simulink model "BreakerFeederFault"  (R2019a)
settings: Solver=ode1  StartTime=0.0  StopTime=2.5  FixedStep=Ts_Power  RelTol=1e-3
PostLoadFcn:
  | %% Init for wind PnO models - global system parameters
  | OVERRIDE_SSN_MEMORY_LIMIT=1;
  | Ts=50e-6;
  | % Ts=50e-10;
  | Ts_Power=Ts;
  | Ts_Control=2*Ts;
  | freq = 50;
  | Fnom=freq;
  | Vac=400e3;
InitFcn:
  | %% Init for wind PnO models - global system parameters
  | OVERRIDE_SSN_MEMORY_LIMIT=1;
  | Ts=50e-6;
  | % Ts=50e-10;
  | Ts_Power=Ts;
  | Ts_Control=2*Ts;
  | freq = 50;
  | Fnom=freq;
  | Vac=225e3;
values from neighbouring files (symbols this model uses):
  ohl_posCap = (0.01e-006)*12    (= 1.2e-07)    [variable.m]
  ohl_posInd = (1.15e-3)/12    (= 9.58333333333e-05)    [variable.m]
  ohl_posR = 0.069/12    (= 0.00575)    [variable.m]
  ohl_zeroCap = (0.004e-006)*12    (= 4.8e-08)    [variable.m]
  ohl_zeroInd = (2.86e-3)/12    (= 0.000238333333333)    [variable.m]
  ohl_zeroR = 0.1725/12    (= 0.014375)    [variable.m]
  sub_Ind = compensate_power    (= 870283996.897)    [variable.m]
  sub_posCap = sub_posCap*6    (= 9.6e-07)    [variable.m]
  sub_posInd = sub_posInd/6    (= 0.000233333333333)    [variable.m]
  sub_posR = sub_posR/6    (= 0.006)    [variable.m]
  sub_zeroCap = sub_zeroCap*6    (= 3.84e-07)    [variable.m]
  sub_zeroInd = sub_zeroInd/6    (= 0.000583333333333)    [variable.m]
  sub_zeroR = sub_zeroR/6    (= 0.015)    [variable.m]
  transfo_L1 = 0.05999374    [variable.m]
  transfo_L2 = 0.05999374    [variable.m]
  transfo_R1 = 0.000866667    [variable.m]
  transfo_R2 = 0.00086667    [variable.m]
undefined symbols (not defined in the file or in its folder): D1, D11, Delta, den, DiscIntNeverNeededParam, dx, find_system, gcbh, num, out_Buses, out_WindFarms, sps_rtmsupport
libraries: powerlib x209, simulink x96, powerlib_meascontrol x96, elements x52, eeSinusoidalMeasurement x51, simulink_extras x42, spsVIMeasurementModel x36, eePowerMeasurement x16
(part 8 of 24)

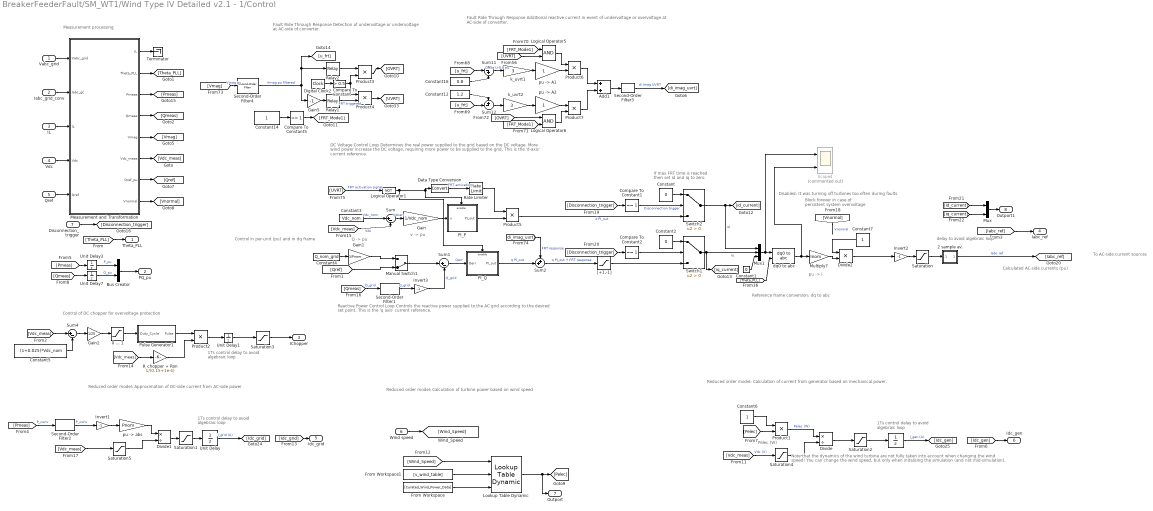
== system BreakerFeederFault/SM_WT1/Wind Type IV Detailed v2.1 - 1/Control ==
  note: Pelec (W)
  note: Note that the dynamics of the wind turbine are not fully taken into account when changing the wind speed! You can change the wind speed, but only when initalising the simulation (and not mid-simulation).
  note: 1Ts control delay to
      | avoid algebraic loop
  note: Reduced order model: Calculation of turbine power based on wind speed
  note: Block forever in case of
      | persistent system overvoltage
  note: 1Ts control delay to
      | avoid algebraic loop
  note: delay to avoid
      |  algebraic loop
  note: Reduced order model: Calculation of current from generator based on mechanical power.
  note: Reduced order model: Approximation of DC-side current from AC-side power
  note: 1Ts control delay to
      | avoid algebraic loop
  note: Reference frame conversion: dq to abc
  note: Control in per-unit (pu) and in dq frame
  note: v -> pu
  note: Reactive Power Control Loop
      | Controls the reactive power supplied to the AC grid according to the desired set point. This is the 'q axis' current reference.
  note: DC Voltage Control Loop
      | Determines the real power supplied to the grid based on the DC voltage. More wind power increase the DC voltage, requiring more power to be supplied to the grid. This is the 'd-axis' current reference.
  note: To AC-side current sources
  note: Q -> pu
  note: pu -> i
  note: Calculated AC-side currents (pu)
  note: Fault Ride Through Response
      | Detection of undervoltage or undervoltage at AC-side of converter.
  note: Fault Ride Through Response
      | Additional reactive current in event of undervoltage or overvoltage at AC-side of converter.
  note: Control of DC chopper for overvoltage protection
  note: Measurement processing
  note: If max FRT time is reached
      | then set id and iq to zero
  note: Disabled: It was turning off turbines too often during faults
  Vabc_grid : Inport
  Iabc_grid_conv : Inport  Port=2
  IL : Inport  Port=3
  Vdc : Inport  Port=4
  Qref : Inport  Port=5
  Wind speed : Inport  Port=6
  Disconnection_trigger : Inport  Port=7
  " " : UnitDelay  SampleTime=-1  HasFrameUpgradeWarning=on
  0 ... 1 : Saturate  UpperLimit=1  LowerLimit=0
  2 sample av. : Subsystem  mask{Init_value=0, Ts=Ts}
      mask prompts: Init_value "Initial value:"; Ts "Sample time (Ts):"
  Add1 : Sum
  Bus Creator : BusCreator  Inputs=2
  Compare To Constant : simulink/Logic and Bit Operations/Compare To Constant  relop=>  const=0.5  OutDataTypeStr=boolean
  Compare To Constant1 : simulink/Logic and Bit Operations/Compare To Constant  relop===  const=1  OutDataTypeStr=boolean
  Compare To Constant2 : simulink/Logic and Bit Operations/Compare To Constant  relop===  const=1  OutDataTypeStr=boolean
  Compare To Constant5 : simulink/Logic and Bit Operations/Compare To Constant  relop===  const=1  OutDataTypeStr=boolean
  Constant : Constant  Value=0
  Constant1 : Constant  Value=0  OutDataTypeStr=Inherit: Inherit via back propagation
  Constant12 : Constant  Value=1.2  SampleTime=Ts
  Constant14 : Constant  SampleTime=Ts
  Constant16 : Constant  Value=0.8  SampleTime=Ts
  Constant2 : Constant  Value=0
  Constant3 : Constant  Value=Vdc_nom
  Constant4 : Constant  Value=Q_nom_grid
  Constant5 : Constant  Value=(1+0.025)*Vdc_nom  SampleTime=Ts
  Constant6 : Constant
  Constant7 : Constant
  Data Type Conversion : DataTypeConversion
  Digital Clock2 : DigitalClock  SampleTime=Ts
  Divide : Product  Inputs=*/
  Divide1 : Product  Inputs=*/
  Divide2 : Product  Inputs=**
  From Workspace : FromWorkspace  VariableName=[Curated_Wind_Power_Data]  SampleTime=0
  From Workspace1 : FromWorkspace  VariableName=[v_wind_table]  SampleTime=0
  Gain : Gain  Gain=1/Vdc_nom
  Gain1 : Gain  Gain=1/Pnom
  Gain2 : Gain  Gain=1/20
  Gain5 : Gain  Gain=-1
  Invert1 : Gain  Gain=-1
  Invert2 : Gain  Gain=-1
  Invert3 : Gain  Gain=-1
  Logical Operator1 : Logic  Operator=NOT  AllPortsSameDT=off  OutDataTypeStr=boolean
  Logical Operator5 : Logic  AllPortsSameDT=off  OutDataTypeStr=boolean
  Logical Operator6 : Logic  AllPortsSameDT=off  OutDataTypeStr=boolean
  Lookup Table Dynamic : simulink/Lookup Tables/Lookup Table Dynamic  LookUpMeth=Interpolation-Use End Values  OutDataType=fixdt('double')  OutScaling=[]  OutputDataTypeScalingMode=Specify via dialog  OutDataTypeStr=double  DoSatur=off
  Manual Switch1 : ManualSwitch  CurrentSetting=0
  Measurement and Transformation : Subsystem
  Multiply7 : Gain  Gain=Inom
  Mux : Mux  Inputs=2
  Mux1 : Mux  Inputs=3
  PI_P : Subsystem
  PI_Q : Subsystem
  Product{1..7} (7 alike) : Product
  Pulse Generator1 : Subsystem  mask{Freq_sawtooth=Freq_sawtooth, Ts=Ts}
      mask prompts: Freq_sawtooth "Frequency of the carrier (sawtooth signal) (Hz):"; Ts "Sample time (Ts) (s):"
  R_chopper + Ron : Gain  Gain=1/(0.15+1e-4)
  Rate Limiter : RateLimiter  RisingSlewLimit=200  FallingSlewLimit=-100  SampleTimeMode=inherited
  Relay1 : Relay  OnSwitchValue=-(0.7)  OffSwitchValue=-(0.8 + 0.05)  OutDataTypeStr=Inherit: Inherit via back propagation
  Relay2 : Relay  OnSwitchValue=1.2 + 0.05  OffSwitchValue=1.2 - 0.05  OutDataTypeStr=Inherit: Inherit via back propagation
  Saturation : Saturate  UpperLimit=1e6  LowerLimit=-1e6
  Saturation1 : Saturate  UpperLimit=1e6  LowerLimit=-1e6
  Saturation2 : Saturate  UpperLimit=1e6  LowerLimit=-1e6
  Saturation3 : Saturate  UpperLimit=10e3  LowerLimit=-10e3
  Saturation4 : Saturate  UpperLimit=1e6  LowerLimit=10
  Saturation5 : Saturate  UpperLimit=1e6  LowerLimit=10
  Scope4 : Scope  Commented=on  NumInputPorts=2
  Second-Order Filter1 : powerlib_meascontrol/Filters/Second-Order Filter  FilterType=Lowpass  Fo=50  Zeta=0.707  Ts=Ts  Initialize=off  Vac_Init="[0,  0,  60]"  Vdc_Init=0  PlotResponse=off  FreqRange=[0, 500, 1]
      settings: SourceProductBaseCode=PS
  Second-Order Filter2 : powerlib_meascontrol/Filters/Second-Order Filter  FilterType=Lowpass  Fo=50  Zeta=0.707  Ts=Ts  Initialize=off  Vac_Init="[0,  0,  60]"  Vdc_Init=0  PlotResponse=off  FreqRange=[0, 500, 1]
      settings: SourceProductBaseCode=PS
  Second-Order Filter3 : powerlib_meascontrol/Filters/Second-Order Filter  FilterType=Lowpass  Fo=1e3  Zeta=0.707  Ts=Ts  Initialize=off  Vac_Init="[0,  0,  60]"  Vdc_Init=0  PlotResponse=off  FreqRange=[0, 500, 1]
      settings: SourceProductBaseCode=PS
  Second-Order Filter4 : powerlib_meascontrol/Filters/Second-Order Filter  FilterType=Lowpass  Fo=100  Zeta=0.707  Ts=Ts  Initialize=off  Vac_Init="[0,  0,  60]"  Vdc_Init=0  PlotResponse=off  FreqRange=[0, 500, 1]
      settings: SourceProductBaseCode=PS
  Sum : Sum  Inputs=|+-
  Sum1 : Sum  Inputs=|+-
  Sum11 : Sum  Inputs=|-+
  Sum12 : Sum  Inputs=+-|
  Sum2 : Sum  Inputs=++|
  Sum4 : Sum  Inputs=|+-
  Switch1 : Switch  Criteria=u2 > Threshold
  Switch2 : Switch  Criteria=u2 > Threshold
  Terminator : Terminator
  Unit Delay : UnitDelay  SampleTime=-1  HasFrameUpgradeWarning=on
  Unit Delay1 : UnitDelay  SampleTime=Ts  HasFrameUpgradeWarning=on
  Unit Delay3 : UnitDelay  SampleTime=Ts  HasFrameUpgradeWarning=on
  Unit Delay7 : UnitDelay  SampleTime=Ts  HasFrameUpgradeWarning=on
  "[+1,-1]" : Saturate  UpperLimit=1  LowerLimit=-1
  dq0 to abc : powerlib_meascontrol/Transformations/dq0 to abc  Alignment=90 degrees behind phase A axis
  k_uvrt1 : Gain  Gain=3
  k_uvrt2 : Gain  Gain=3
  "pu -> A1" : Gain
  "pu -> A2" : Gain
  "pu -> abs" : Gain  Gain=Pnom
  Theta_PLL : Outport  VectorParamsAs1DForOutWhenUnconnected=on
  PQ_pu : Outport  Port=2  VectorParamsAs1DForOutWhenUnconnected=on
  IChopper : Outport  Port=3  VectorParamsAs1DForOutWhenUnconnected=on
  Iabc_ref : Outport  Port=4  VectorParamsAs1DForOutWhenUnconnected=on
  Idc_grid : Outport  Port=5  VectorParamsAs1DForOutWhenUnconnected=on
  Idc_gen : Outport  Port=6  VectorParamsAs1DForOutWhenUnconnected=on
  Outport : Outport  Port=7  VectorParamsAs1DForOutWhenUnconnected=on
  Outport1 : Outport  Port=8  VectorParamsAs1DForOutWhenUnconnected=on
  wires:
  Constant7/1 -> Divide2/1
  Disconnection_trigger/1 -> [Disconnection_trigger]
  Mux/1 -> Outport1/1
  [iq_current] -> Mux/2
  [id_current] -> Mux/1
  Compare To Constant2/1 -> Switch1/2
  [Disconnection_trigger] -> Compare To Constant2/1
  Compare To Constant1/1 -> Switch2/2  "Disconnection trigger"
  [Disconnection_trigger] -> Compare To Constant1/1
  "[+1,-1]"/1 -> Switch1/3
  Constant2/1 -> Switch1/1
  Product5/1 -> Switch2/3  "d PI_out"
  Constant/1 -> Switch2/1
  Switch1/1 -> Mux1/2, [iq_current]  "iq"
  Switch2/1 -> [id_current], Mux1/1  "id"
  From Workspace/1 -> Lookup Table Dynamic/3
  From Workspace1/1 -> Lookup Table Dynamic/2
  [Wind_Speed] -> Lookup Table Dynamic/1
  Lookup Table Dynamic/1 -> [Pelec], Outport/1
  Logical Operator1/1 -> PI_Q/Enable, PI_P/Enable, Data Type Conversion/1
  [UVRT] -> Logical Operator1/1  "FRT activation signal"
  [di_imag_uvrt] -> Sum2/1  "FRT response"
  Sum2/1 -> "[+1,-1]"/1  "q PI_out + FRT response"
  Second-Order Filter3/1 -> [di_imag_uvrt]  "di Imag UVRT"
  2 sample av./1(out) -> [Iabc_ref]  "Iabc ref"
  [Iabc_ref] -> Iabc_ref/1
  Product6/1 -> Add1/1
  " "/1 -> [Idc_gen]  "I_gen (A)"
  Product1/1 -> Divide/1  "Pelec (W)"
  [Pelec] -> Product1/2
  [Idc_gen] -> Idc_gen/1
  Constant6/1 -> Product1/1
  [Vdc_meas] -> Saturation4/1  "Vdc (V)"
  Saturation2/1 -> " "/1
  Divide/1 -> Saturation2/1
  Saturation4/1 -> Divide/2
  Wind speed/1 -> [Wind_Speed]
  [Vnormal] -> ?  "Vnormal"
  Divide2/1 -> Invert2/1
  Measurement and Transformation/8(Vnormal) -> [Vnormal]
  PI_Q/1(PI_out) -> Sum2/2  "q PI_out"
  Saturation5/1 -> Divide1/2
  Saturation1/1 -> Unit Delay/1
  Saturation/1 -> 2 sample av./1(in)
  PI_P/1(PI_out) -> Product5/2
  Gain/1 -> PI_P/1(u)
  Rate Limiter/1 -> Product5/1
  Constant4/1 -> Gain1/1
  [Pmeas] -> Second-Order Filter2/1  "P_conv"
  [Qmeas] -> Second-Order Filter1/1  "Q_grid"
  Second-Order Filter1/1 -> Invert3/1  "Q_grid"
  Saturation3/1 -> IChopper/1
  Invert2/1 -> Saturation/1
  [Idc_grid] -> Idc_grid/1
  [Vdc_meas] -> Saturation5/1
  Second-Order Filter2/1 -> Invert1/1  "P_conv"
  Unit Delay/1 -> [Idc_grid]  "I_grid (A)"
  Divide1/1 -> Saturation1/1
  Invert1/1 -> "pu -> abs"/1
  "pu -> abs"/1 -> Divide1/1
  Measurement and Transformation/7(Qref_pu) -> [Qref]
  Sum/1 -> Gain/1  "Vdcerr"
  [Theta_PLL] -> dq0 to abc/2
  Sum1/1 -> PI_Q/1(Qerr)  "Qerr"
  Constant3/1 -> Sum/1  "Vdc_nom"
  Invert3/1 -> Sum1/2  "Q_grid"
  [Vdc_meas] -> Sum/2  "Vdc"
  Mux1/1 -> dq0 to abc/1, Scope4/1
  Manual Switch1/1 -> Sum1/1
  dq0 to abc/1 -> Multiply7/1, Scope4/2
  Constant1/1 -> Mux1/3
  Data Type Conversion/1 -> Rate Limiter/1  "FRT activation"
  Gain1/1 -> Manual Switch1/1
  Multiply7/1 -> Divide2/2
  [Qref] -> Manual Switch1/2
  Relay1/1 -> Product4/2  "FRT triggered"
  "pu -> A2"/1 -> Product7/1
  [FRT_Mode1] -> Logical Operator5/1
  k_uvrt1/1 -> "pu -> A1"/1
  [FRT_Mode1] -> Logical Operator6/2
  Sum12/1 -> k_uvrt2/1
  [Vmag] -> Second-Order Filter4/1  "Vmag pu"
  k_uvrt2/1 -> "pu -> A2"/1
  Gain5/1 -> Relay1/1
  [OVRT] -> Logical Operator6/1
  Logical Operator5/1 -> Product6/1
  Sum11/1 -> k_uvrt1/1  "Delta U-0.8 pu"
  Logical Operator6/1 -> Product7/2
  Second-Order Filter4/1 -> Gain5/1, Relay2/1, [u_frt]  "Vmag pu filtered"
  Constant16/1 -> Sum11/2
  Product3/1 -> [OVRT]
  Digital Clock2/1 -> Compare To Constant/1
  Add1/1 -> Second-Order Filter3/1
  Product4/1 -> [UVRT]
  Relay2/1 -> Product3/1
  Product7/1 -> Add1/2
  "pu -> A1"/1 -> Product6/2
  Compare To Constant/1 -> Product3/2, Product4/1
  [UVRT] -> Logical Operator5/2
  [u_frt] -> Sum12/2
  Constant12/1 -> Sum12/1
  Compare To Constant5/1 -> [FRT_Mode1]
  [u_frt] -> Sum11/1
  Constant14/1 -> Compare To Constant5/1
  Unit Delay1/1 -> Saturation3/1
  Pulse Generator1/1(Pulse) -> Product2/1
  [Vdc_meas] -> R_chopper + Ron/1
  Product2/1 -> Unit Delay1/1
  R_chopper + Ron/1 -> Product2/2
  Measurement and Transformation/6(Vdc_meas) -> [Vdc_meas]
  0 ... 1/1 -> Pulse Generator1/1(Duty_Cycle)
  Gain2/1 -> 0 ... 1/1
  Sum4/1 -> Gain2/1
  [Vdc_meas] -> Sum4/1
  Constant5/1 -> Sum4/2
  Measurement and Transformation/5(Vmag) -> [Vmag]
  Measurement and Transformation/4(Qmeas) -> [Qmeas]
  Measurement and Transformation/3(Pmeas) -> [Pmeas]
  [Theta_PLL] -> Theta_PLL/1
  Vabc_grid/1 -> Measurement and Transformation/1(Vabc_grid)
  Iabc_grid_conv/1 -> Measurement and Transformation/2(Iabc_gc)
  IL/1 -> Measurement and Transformation/3(IL)
  Qref/1 -> Measurement and Transformation/5(Qref)
  Measurement and Transformation/2(Theta_PLL) -> [Theta_PLL]
  Measurement and Transformation/1("IL ") -> Terminator/1
  Vdc/1 -> Measurement and Transformation/4(Vdc)
  [Pmeas] -> Unit Delay3/1
  [Qmeas] -> Unit Delay7/1
  Unit Delay7/1 -> Bus Creator/2  "Q_pu"
  Unit Delay3/1 -> Bus Creator/1  "P_pu"
  Bus Creator/1 -> PQ_pu/1

== system BreakerFeederFault/SM_WT1/Wind Type IV Detailed v2.1 - 2/AC fault ride though characteristic ==
  note: If more than X seconds under
      | FRT then disconnection message
  Va pu mag : Inport
  I 3ph pu : Inport  Port=2
  Compare To Constant : simulink/Logic and Bit Operations/Compare To Constant  relop=>=  const=Fault_Base_Duration_time_FRT  OutDataTypeStr=boolean
  Compare To Constant1 : simulink/Logic and Bit Operations/Compare To Constant  relop=<  const=0.2  OutDataTypeStr=boolean
  Compare To Constant2 : simulink/Logic and Bit Operations/Compare To Constant  relop=<  const=0.2  OutDataTypeStr=boolean
  Compare To Constant3 : simulink/Logic and Bit Operations/Compare To Constant  relop=<  const=0.5  OutDataTypeStr=boolean
  Constant : Constant  Value=0  SampleTime=Ts
  Constant1 : Constant  SampleTime=Ts
  Constant2 : Constant  Value=0  SampleTime=Ts
  Constant3 : Constant  Value=0
  Constant4 : Constant  Value=0
  Constant5 : Constant  Value=0
  Constant6 : Constant  Value=0.9  SampleTime=Ts
  Data Type Conversion : DataTypeConversion  OutDataTypeStr=double
  Digital Clock{1..4} (4 alike) : DigitalClock  SampleTime=Ts
  Discrete-Time Integrator : DiscreteIntegrator  ExternalReset=rising  SampleTime=Ts  ICPrevOutput=DiscIntNeverNeededParam  ICPrevScaledInput=DiscIntNeverNeededParam
  Memory : Memory
  MinMax : MinMax  Function=max
  MinMax Running Resettable : simulink/Math Operations/MinMax Running Resettable  Function=max  vinit=0.0
  MinMax Running Resettable1 : simulink/Math Operations/MinMax Running Resettable  Function=min  vinit=1
  MinMax Running Resettable2 : simulink/Math Operations/MinMax Running Resettable  Function=max  vinit=0.0
  MinMax1 : MinMax  Function=max
  MinMax2 : MinMax
  NOT : Logic  Operator=NOT  AllPortsSameDT=off  OutDataTypeStr=boolean
  OR : Logic  Operator=OR  AllPortsSameDT=off  OutDataTypeStr=boolean
  Relational Operator : RelationalOperator  Operator=<  OutDataTypeStr=boolean  RndMeth=Simplest
  "Sinusoidal Measurement (PLL, Three-Phase)1" : eeSinusoidalMeasurement/Sinusoidal Measurement (PLL, Three-Phase)  Kp_LF=200  Ki_LF=2000  F0=freq  Theta0=0  Ts=Ts
      settings: SourceProductBaseCode=PS
  Switch1 : Switch  Criteria=u2 > Threshold
  Switch2 : Switch  Criteria=u2 > Threshold
  Switch3 : Switch  Criteria=u2 > Threshold
  Terminator : Terminator
  Terminator1 : Terminator
  Triggered Subsystem : Subsystem  TreatAsAtomicUnit=on
  Disconnection_trigger : Outport  VectorParamsAs1DForOutWhenUnconnected=on
  Time_under_FRT : Outport  Port=2  VectorParamsAs1DForOutWhenUnconnected=on
  Min_voltage : Outport  Port=3  VectorParamsAs1DForOutWhenUnconnected=on
  Max_current : Outport  Port=4  VectorParamsAs1DForOutWhenUnconnected=on
  Time_trigger_FRT : Outport  Port=5  VectorParamsAs1DForOutWhenUnconnected=on
  wires:
  Constant6/1 -> Relational Operator/2
  Discrete-Time Integrator/1 -> Compare To Constant/1, MinMax/1  "Integrator output"
  Digital Clock1/1 -> Compare To Constant3/1
  Relational Operator/1 -> Switch2/3
  Compare To Constant3/1 -> Switch2/2
  Constant/1 -> Switch2/1
  Switch2/1 -> NOT/1, Discrete-Time Integrator/1  "Va comparison to Vgrid"
  NOT/1 -> Discrete-Time Integrator/2
  OR/1 -> Triggered Subsystem/Trigger, Data Type Conversion/1, Memory/1  "Disconnection_Trigger"
  Compare To Constant/1 -> OR/2
  Memory/1 -> OR/1
  MinMax/1 -> MinMax Running Resettable/1
  MinMax Running Resettable/1 -> Time_under_FRT/1
  Va pu mag/1 -> Relational Operator/1, Switch3/3
  MinMax1/1 -> MinMax Running Resettable2/1
  MinMax Running Resettable2/1 -> Max_current/1
  I 3ph pu/1 -> "Sinusoidal Measurement (PLL, Three-Phase)1"/1
  "Sinusoidal Measurement (PLL, Three-Phase)1"/3 -> Switch1/3  "Vabc_pu_mag"
  "Sinusoidal Measurement (PLL, Three-Phase)1"/2 -> Terminator/1
  "Sinusoidal Measurement (PLL, Three-Phase)1"/1 -> Terminator1/1
  MinMax Running Resettable1/1 -> Min_voltage/1
  Compare To Constant1/1 -> Switch3/2
  Constant1/1 -> Switch3/1
  Digital Clock2/1 -> Compare To Constant1/1
  Digital Clock3/1 -> Triggered Subsystem/1(In1)
  Triggered Subsystem/1(Time_trigger_FRT) -> Time_trigger_FRT/1
  Digital Clock4/1 -> Compare To Constant2/1
  Constant2/1 -> Switch1/1
  Compare To Constant2/1 -> Switch1/2
  Switch1/1 -> MinMax1/1
  Switch3/1 -> MinMax2/1
  MinMax2/1 -> MinMax Running Resettable1/1
  Constant3/1 -> MinMax Running Resettable/2
  Constant4/1 -> MinMax Running Resettable1/2
  Constant5/1 -> MinMax Running Resettable2/2
  Data Type Conversion/1 -> Disconnection_trigger/1

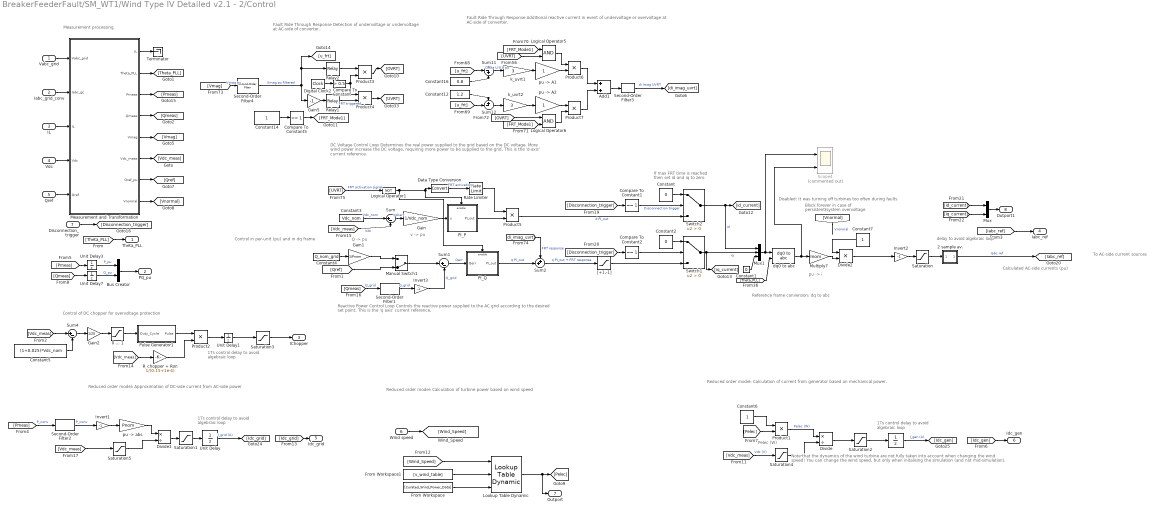
== system BreakerFeederFault/SM_WT1/Wind Type IV Detailed v2.1 - 2/Control ==
  note: Disabled: It was turning off turbines too often during faults
  note: If max FRT time is reached
      | then set id and iq to zero
  note: Measurement processing
  note: Control of DC chopper for overvoltage protection
  note: Fault Ride Through Response
      | Additional reactive current in event of undervoltage or overvoltage at AC-side of converter.
  note: Fault Ride Through Response
      | Detection of undervoltage or undervoltage at AC-side of converter.
  note: Calculated AC-side currents (pu)
  note: pu -> i
  note: Q -> pu
  note: To AC-side current sources
  note: DC Voltage Control Loop
      | Determines the real power supplied to the grid based on the DC voltage. More wind power increase the DC voltage, requiring more power to be supplied to the grid. This is the 'd-axis' current reference.
  note: Reactive Power Control Loop
      | Controls the reactive power supplied to the AC grid according to the desired set point. This is the 'q axis' current reference.
  note: v -> pu
  note: Control in per-unit (pu) and in dq frame
  note: Reference frame conversion: dq to abc
  note: 1Ts control delay to
      | avoid algebraic loop
  note: Reduced order model: Approximation of DC-side current from AC-side power
  note: Reduced order model: Calculation of current from generator based on mechanical power.
  note: delay to avoid
      |  algebraic loop
  note: 1Ts control delay to
      | avoid algebraic loop
  note: Block forever in case of
      | persistent system overvoltage
  note: Reduced order model: Calculation of turbine power based on wind speed
  note: 1Ts control delay to
      | avoid algebraic loop
  note: Note that the dynamics of the wind turbine are not fully taken into account when changing the wind speed! You can change the wind speed, but only when initalising the simulation (and not mid-simulation).
  note: Pelec (W)
  Vabc_grid : Inport
  Iabc_grid_conv : Inport  Port=2
  IL : Inport  Port=3
  Vdc : Inport  Port=4
  Qref : Inport  Port=5
  Wind speed : Inport  Port=6
  Disconnection_trigger : Inport  Port=7
  " " : UnitDelay  SampleTime=-1  HasFrameUpgradeWarning=on
  0 ... 1 : Saturate  UpperLimit=1  LowerLimit=0
  2 sample av. : Subsystem  mask{Init_value=0, Ts=Ts}
      mask prompts: Init_value "Initial value:"; Ts "Sample time (Ts):"
  Add1 : Sum
  Bus Creator : BusCreator  Inputs=2
  Compare To Constant : simulink/Logic and Bit Operations/Compare To Constant  relop=>  const=0.5  OutDataTypeStr=boolean
  Compare To Constant1 : simulink/Logic and Bit Operations/Compare To Constant  relop===  const=1  OutDataTypeStr=boolean
  Compare To Constant2 : simulink/Logic and Bit Operations/Compare To Constant  relop===  const=1  OutDataTypeStr=boolean
  Compare To Constant5 : simulink/Logic and Bit Operations/Compare To Constant  relop===  const=1  OutDataTypeStr=boolean
  Constant : Constant  Value=0
  Constant1 : Constant  Value=0  OutDataTypeStr=Inherit: Inherit via back propagation
  Constant12 : Constant  Value=1.2  SampleTime=Ts
  Constant14 : Constant  SampleTime=Ts
  Constant16 : Constant  Value=0.8  SampleTime=Ts
  Constant2 : Constant  Value=0
  Constant3 : Constant  Value=Vdc_nom
  Constant4 : Constant  Value=Q_nom_grid
  Constant5 : Constant  Value=(1+0.025)*Vdc_nom  SampleTime=Ts
  Constant6 : Constant
  Constant7 : Constant
  Data Type Conversion : DataTypeConversion
  Digital Clock2 : DigitalClock  SampleTime=Ts
  Divide : Product  Inputs=*/
  Divide1 : Product  Inputs=*/
  Divide2 : Product  Inputs=**
  From Workspace : FromWorkspace  VariableName=[Curated_Wind_Power_Data]  SampleTime=0
  From Workspace1 : FromWorkspace  VariableName=[v_wind_table]  SampleTime=0
  Gain : Gain  Gain=1/Vdc_nom
  Gain1 : Gain  Gain=1/Pnom
  Gain2 : Gain  Gain=1/20
  Gain5 : Gain  Gain=-1
  Invert1 : Gain  Gain=-1
  Invert2 : Gain  Gain=-1
  Invert3 : Gain  Gain=-1
  Logical Operator1 : Logic  Operator=NOT  AllPortsSameDT=off  OutDataTypeStr=boolean
  Logical Operator5 : Logic  AllPortsSameDT=off  OutDataTypeStr=boolean
  Logical Operator6 : Logic  AllPortsSameDT=off  OutDataTypeStr=boolean
  Lookup Table Dynamic : simulink/Lookup Tables/Lookup Table Dynamic  LookUpMeth=Interpolation-Use End Values  OutDataType=fixdt('double')  OutScaling=[]  OutputDataTypeScalingMode=Specify via dialog  OutDataTypeStr=double  DoSatur=off
  Manual Switch1 : ManualSwitch  CurrentSetting=0
  Measurement and Transformation : Subsystem
  Multiply7 : Gain  Gain=Inom
  Mux : Mux  Inputs=2
  Mux1 : Mux  Inputs=3
  PI_P : Subsystem
  PI_Q : Subsystem
  Product{1..7} (7 alike) : Product
  Pulse Generator1 : Subsystem  mask{Freq_sawtooth=Freq_sawtooth, Ts=Ts}
      mask prompts: Freq_sawtooth "Frequency of the carrier (sawtooth signal) (Hz):"; Ts "Sample time (Ts) (s):"
  R_chopper + Ron : Gain  Gain=1/(0.15+1e-4)
  Rate Limiter : RateLimiter  RisingSlewLimit=200  FallingSlewLimit=-100  SampleTimeMode=inherited
  Relay1 : Relay  OnSwitchValue=-(0.7)  OffSwitchValue=-(0.8 + 0.05)  OutDataTypeStr=Inherit: Inherit via back propagation
  Relay2 : Relay  OnSwitchValue=1.2 + 0.05  OffSwitchValue=1.2 - 0.05  OutDataTypeStr=Inherit: Inherit via back propagation
  Saturation : Saturate  UpperLimit=1e6  LowerLimit=-1e6
  Saturation1 : Saturate  UpperLimit=1e6  LowerLimit=-1e6
  Saturation2 : Saturate  UpperLimit=1e6  LowerLimit=-1e6
  Saturation3 : Saturate  UpperLimit=10e3  LowerLimit=-10e3
  Saturation4 : Saturate  UpperLimit=1e6  LowerLimit=10
  Saturation5 : Saturate  UpperLimit=1e6  LowerLimit=10
  Scope4 : Scope  Commented=on  NumInputPorts=2
  Second-Order Filter1 : powerlib_meascontrol/Filters/Second-Order Filter  FilterType=Lowpass  Fo=50  Zeta=0.707  Ts=Ts  Initialize=off  Vac_Init="[0,  0,  60]"  Vdc_Init=0  PlotResponse=off  FreqRange=[0, 500, 1]
      settings: SourceProductBaseCode=PS
  Second-Order Filter2 : powerlib_meascontrol/Filters/Second-Order Filter  FilterType=Lowpass  Fo=50  Zeta=0.707  Ts=Ts  Initialize=off  Vac_Init="[0,  0,  60]"  Vdc_Init=0  PlotResponse=off  FreqRange=[0, 500, 1]
      settings: SourceProductBaseCode=PS
  Second-Order Filter3 : powerlib_meascontrol/Filters/Second-Order Filter  FilterType=Lowpass  Fo=1e3  Zeta=0.707  Ts=Ts  Initialize=off  Vac_Init="[0,  0,  60]"  Vdc_Init=0  PlotResponse=off  FreqRange=[0, 500, 1]
      settings: SourceProductBaseCode=PS
  Second-Order Filter4 : powerlib_meascontrol/Filters/Second-Order Filter  FilterType=Lowpass  Fo=100  Zeta=0.707  Ts=Ts  Initialize=off  Vac_Init="[0,  0,  60]"  Vdc_Init=0  PlotResponse=off  FreqRange=[0, 500, 1]
      settings: SourceProductBaseCode=PS
  Sum : Sum  Inputs=|+-
  Sum1 : Sum  Inputs=|+-
  Sum11 : Sum  Inputs=|-+
  Sum12 : Sum  Inputs=+-|
  Sum2 : Sum  Inputs=++|
  Sum4 : Sum  Inputs=|+-
  Switch1 : Switch  Criteria=u2 > Threshold
  Switch2 : Switch  Criteria=u2 > Threshold
  Terminator : Terminator
  Unit Delay : UnitDelay  SampleTime=-1  HasFrameUpgradeWarning=on
  Unit Delay1 : UnitDelay  SampleTime=Ts  HasFrameUpgradeWarning=on
  Unit Delay3 : UnitDelay  SampleTime=Ts  HasFrameUpgradeWarning=on
  Unit Delay7 : UnitDelay  SampleTime=Ts  HasFrameUpgradeWarning=on
  "[+1,-1]" : Saturate  UpperLimit=1  LowerLimit=-1
  dq0 to abc : powerlib_meascontrol/Transformations/dq0 to abc  Alignment=90 degrees behind phase A axis
  k_uvrt1 : Gain  Gain=3
  k_uvrt2 : Gain  Gain=3
  "pu -> A1" : Gain
  "pu -> A2" : Gain
  "pu -> abs" : Gain  Gain=Pnom
  Theta_PLL : Outport  VectorParamsAs1DForOutWhenUnconnected=on
  PQ_pu : Outport  Port=2  VectorParamsAs1DForOutWhenUnconnected=on
  IChopper : Outport  Port=3  VectorParamsAs1DForOutWhenUnconnected=on
  Iabc_ref : Outport  Port=4  VectorParamsAs1DForOutWhenUnconnected=on
  Idc_grid : Outport  Port=5  VectorParamsAs1DForOutWhenUnconnected=on
  Idc_gen : Outport  Port=6  VectorParamsAs1DForOutWhenUnconnected=on
  Outport : Outport  Port=7  VectorParamsAs1DForOutWhenUnconnected=on
  Outport1 : Outport  Port=8  VectorParamsAs1DForOutWhenUnconnected=on
  wires:
  Bus Creator/1 -> PQ_pu/1
  Unit Delay3/1 -> Bus Creator/1  "P_pu"
  Unit Delay7/1 -> Bus Creator/2  "Q_pu"
  [Qmeas] -> Unit Delay7/1
  [Pmeas] -> Unit Delay3/1
  Vdc/1 -> Measurement and Transformation/4(Vdc)
  Measurement and Transformation/1("IL ") -> Terminator/1
  Measurement and Transformation/2(Theta_PLL) -> [Theta_PLL]
  Qref/1 -> Measurement and Transformation/5(Qref)
  IL/1 -> Measurement and Transformation/3(IL)
  Iabc_grid_conv/1 -> Measurement and Transformation/2(Iabc_gc)
  Vabc_grid/1 -> Measurement and Transformation/1(Vabc_grid)
  [Theta_PLL] -> Theta_PLL/1
  Measurement and Transformation/3(Pmeas) -> [Pmeas]
  Measurement and Transformation/4(Qmeas) -> [Qmeas]
  Measurement and Transformation/5(Vmag) -> [Vmag]
  Constant5/1 -> Sum4/2
  [Vdc_meas] -> Sum4/1
  Sum4/1 -> Gain2/1
  Gain2/1 -> 0 ... 1/1
  0 ... 1/1 -> Pulse Generator1/1(Duty_Cycle)
  Measurement and Transformation/6(Vdc_meas) -> [Vdc_meas]
  R_chopper + Ron/1 -> Product2/2
  Product2/1 -> Unit Delay1/1
  [Vdc_meas] -> R_chopper + Ron/1
  Pulse Generator1/1(Pulse) -> Product2/1
  Unit Delay1/1 -> Saturation3/1
  Constant14/1 -> Compare To Constant5/1
  [u_frt] -> Sum11/1
  Compare To Constant5/1 -> [FRT_Mode1]
  Constant12/1 -> Sum12/1
  [u_frt] -> Sum12/2
  [UVRT] -> Logical Operator5/2
  Compare To Constant/1 -> Product4/1, Product3/2
  "pu -> A1"/1 -> Product6/2
  Product7/1 -> Add1/2
  Relay2/1 -> Product3/1
  Product4/1 -> [UVRT]
  Add1/1 -> Second-Order Filter3/1
  Digital Clock2/1 -> Compare To Constant/1
  Product3/1 -> [OVRT]
  Constant16/1 -> Sum11/2
  Second-Order Filter4/1 -> [u_frt], Relay2/1, Gain5/1  "Vmag pu filtered"
  Logical Operator6/1 -> Product7/2
  Sum11/1 -> k_uvrt1/1  "Delta U-0.8 pu"
  Logical Operator5/1 -> Product6/1
  [OVRT] -> Logical Operator6/1
  Gain5/1 -> Relay1/1
  k_uvrt2/1 -> "pu -> A2"/1
  [Vmag] -> Second-Order Filter4/1  "Vmag pu"
  Sum12/1 -> k_uvrt2/1
  [FRT_Mode1] -> Logical Operator6/2
  k_uvrt1/1 -> "pu -> A1"/1
  [FRT_Mode1] -> Logical Operator5/1
  "pu -> A2"/1 -> Product7/1
  Relay1/1 -> Product4/2  "FRT triggered"
  [Qref] -> Manual Switch1/2
  Multiply7/1 -> Divide2/2
  Gain1/1 -> Manual Switch1/1
  Data Type Conversion/1 -> Rate Limiter/1  "FRT activation"
  Constant1/1 -> Mux1/3
  dq0 to abc/1 -> Scope4/2, Multiply7/1
  Manual Switch1/1 -> Sum1/1
  Mux1/1 -> Scope4/1, dq0 to abc/1
  [Vdc_meas] -> Sum/2  "Vdc"
  Invert3/1 -> Sum1/2  "Q_grid"
  Constant3/1 -> Sum/1  "Vdc_nom"
  Sum1/1 -> PI_Q/1(Qerr)  "Qerr"
  [Theta_PLL] -> dq0 to abc/2
  Sum/1 -> Gain/1  "Vdcerr"
  Measurement and Transformation/7(Qref_pu) -> [Qref]
  "pu -> abs"/1 -> Divide1/1
  Invert1/1 -> "pu -> abs"/1
  Divide1/1 -> Saturation1/1
  Unit Delay/1 -> [Idc_grid]  "I_grid (A)"
  Second-Order Filter2/1 -> Invert1/1  "P_conv"
  [Vdc_meas] -> Saturation5/1
  [Idc_grid] -> Idc_grid/1
  Invert2/1 -> Saturation/1
  Saturation3/1 -> IChopper/1
  Second-Order Filter1/1 -> Invert3/1  "Q_grid"
  [Qmeas] -> Second-Order Filter1/1  "Q_grid"
  [Pmeas] -> Second-Order Filter2/1  "P_conv"
  Constant4/1 -> Gain1/1
  Rate Limiter/1 -> Product5/1
  Gain/1 -> PI_P/1(u)
  PI_P/1(PI_out) -> Product5/2
  Saturation/1 -> 2 sample av./1(in)
  Saturation1/1 -> Unit Delay/1
  Saturation5/1 -> Divide1/2
  PI_Q/1(PI_out) -> Sum2/2  "q PI_out"
  Measurement and Transformation/8(Vnormal) -> [Vnormal]
  Divide2/1 -> Invert2/1
  [Vnormal] -> ?  "Vnormal"
  Wind speed/1 -> [Wind_Speed]
  Saturation4/1 -> Divide/2
  Divide/1 -> Saturation2/1
  Saturation2/1 -> " "/1
  [Vdc_meas] -> Saturation4/1  "Vdc (V)"
  Constant6/1 -> Product1/1
  [Idc_gen] -> Idc_gen/1
  [Pelec] -> Product1/2
  Product1/1 -> Divide/1  "Pelec (W)"
  " "/1 -> [Idc_gen]  "I_gen (A)"
  Product6/1 -> Add1/1
  [Iabc_ref] -> Iabc_ref/1
  2 sample av./1(out) -> [Iabc_ref]  "Iabc ref"
  Second-Order Filter3/1 -> [di_imag_uvrt]  "di Imag UVRT"
  Sum2/1 -> "[+1,-1]"/1  "q PI_out + FRT response"
  [di_imag_uvrt] -> Sum2/1  "FRT response"
  [UVRT] -> Logical Operator1/1  "FRT activation signal"
  Logical Operator1/1 -> Data Type Conversion/1, PI_P/Enable, PI_Q/Enable
  Lookup Table Dynamic/1 -> Outport/1, [Pelec]
  [Wind_Speed] -> Lookup Table Dynamic/1
  From Workspace1/1 -> Lookup Table Dynamic/2
  From Workspace/1 -> Lookup Table Dynamic/3
  Switch2/1 -> Mux1/1, [id_current]  "id"
  Switch1/1 -> [iq_current], Mux1/2  "iq"
  Constant/1 -> Switch2/1
  Product5/1 -> Switch2/3  "d PI_out"
  Constant2/1 -> Switch1/1
  "[+1,-1]"/1 -> Switch1/3
  [Disconnection_trigger] -> Compare To Constant1/1
  Compare To Constant1/1 -> Switch2/2  "Disconnection trigger"
  [Disconnection_trigger] -> Compare To Constant2/1
  Compare To Constant2/1 -> Switch1/2
  [id_current] -> Mux/1
  [iq_current] -> Mux/2
  Mux/1 -> Outport1/1
  Disconnection_trigger/1 -> [Disconnection_trigger]
  Constant7/1 -> Divide2/1

== system BreakerFeederFault/SM_WT1/Wind Type IV Detailed v2.1 - 3/AC fault ride though characteristic ==
  note: If more than X seconds under
      | FRT then disconnection message
  Va pu mag : Inport
  I 3ph pu : Inport  Port=2
  Compare To Constant : simulink/Logic and Bit Operations/Compare To Constant  relop=>=  const=Fault_Base_Duration_time_FRT  OutDataTypeStr=boolean
  Compare To Constant1 : simulink/Logic and Bit Operations/Compare To Constant  relop=<  const=0.2  OutDataTypeStr=boolean
  Compare To Constant2 : simulink/Logic and Bit Operations/Compare To Constant  relop=<  const=0.2  OutDataTypeStr=boolean
  Compare To Constant3 : simulink/Logic and Bit Operations/Compare To Constant  relop=<  const=0.5  OutDataTypeStr=boolean
  Constant : Constant  Value=0  SampleTime=Ts
  Constant1 : Constant  SampleTime=Ts
  Constant2 : Constant  Value=0  SampleTime=Ts
  Constant3 : Constant  Value=0
  Constant4 : Constant  Value=0
  Constant5 : Constant  Value=0
  Constant6 : Constant  Value=0.9  SampleTime=Ts
  Data Type Conversion : DataTypeConversion  OutDataTypeStr=double
  Digital Clock{1..4} (4 alike) : DigitalClock  SampleTime=Ts
  Discrete-Time Integrator : DiscreteIntegrator  ExternalReset=rising  SampleTime=Ts  ICPrevOutput=DiscIntNeverNeededParam  ICPrevScaledInput=DiscIntNeverNeededParam
  Memory : Memory
  MinMax : MinMax  Function=max
  MinMax Running Resettable : simulink/Math Operations/MinMax Running Resettable  Function=max  vinit=0.0
  MinMax Running Resettable1 : simulink/Math Operations/MinMax Running Resettable  Function=min  vinit=1
  MinMax Running Resettable2 : simulink/Math Operations/MinMax Running Resettable  Function=max  vinit=0.0
  MinMax1 : MinMax  Function=max
  MinMax2 : MinMax
  NOT : Logic  Operator=NOT  AllPortsSameDT=off  OutDataTypeStr=boolean
  OR : Logic  Operator=OR  AllPortsSameDT=off  OutDataTypeStr=boolean
  Relational Operator : RelationalOperator  Operator=<  OutDataTypeStr=boolean  RndMeth=Simplest
  "Sinusoidal Measurement (PLL, Three-Phase)1" : eeSinusoidalMeasurement/Sinusoidal Measurement (PLL, Three-Phase)  Kp_LF=200  Ki_LF=2000  F0=freq  Theta0=0  Ts=Ts
      settings: SourceProductBaseCode=PS
  Switch1 : Switch  Criteria=u2 > Threshold
  Switch2 : Switch  Criteria=u2 > Threshold
  Switch3 : Switch  Criteria=u2 > Threshold
  Terminator : Terminator
  Terminator1 : Terminator
  Triggered Subsystem : Subsystem  TreatAsAtomicUnit=on
  Disconnection_trigger : Outport  VectorParamsAs1DForOutWhenUnconnected=on
  Time_under_FRT : Outport  Port=2  VectorParamsAs1DForOutWhenUnconnected=on
  Min_voltage : Outport  Port=3  VectorParamsAs1DForOutWhenUnconnected=on
  Max_current : Outport  Port=4  VectorParamsAs1DForOutWhenUnconnected=on
  Time_trigger_FRT : Outport  Port=5  VectorParamsAs1DForOutWhenUnconnected=on
  wires:
  Constant6/1 -> Relational Operator/2
  Discrete-Time Integrator/1 -> Compare To Constant/1, MinMax/1  "Integrator output"
  Digital Clock1/1 -> Compare To Constant3/1
  Relational Operator/1 -> Switch2/3
  Compare To Constant3/1 -> Switch2/2
  Constant/1 -> Switch2/1
  Switch2/1 -> NOT/1, Discrete-Time Integrator/1  "Va comparison to Vgrid"
  NOT/1 -> Discrete-Time Integrator/2
  OR/1 -> Triggered Subsystem/Trigger, Data Type Conversion/1, Memory/1  "Disconnection_Trigger"
  Compare To Constant/1 -> OR/2
  Memory/1 -> OR/1
  MinMax/1 -> MinMax Running Resettable/1
  MinMax Running Resettable/1 -> Time_under_FRT/1
  Va pu mag/1 -> Relational Operator/1, Switch3/3
  MinMax1/1 -> MinMax Running Resettable2/1
  MinMax Running Resettable2/1 -> Max_current/1
  I 3ph pu/1 -> "Sinusoidal Measurement (PLL, Three-Phase)1"/1
  "Sinusoidal Measurement (PLL, Three-Phase)1"/3 -> Switch1/3  "Vabc_pu_mag"
  "Sinusoidal Measurement (PLL, Three-Phase)1"/2 -> Terminator/1
  "Sinusoidal Measurement (PLL, Three-Phase)1"/1 -> Terminator1/1
  MinMax Running Resettable1/1 -> Min_voltage/1
  Compare To Constant1/1 -> Switch3/2
  Constant1/1 -> Switch3/1
  Digital Clock2/1 -> Compare To Constant1/1
  Digital Clock3/1 -> Triggered Subsystem/1(In1)
  Triggered Subsystem/1(Time_trigger_FRT) -> Time_trigger_FRT/1
  Digital Clock4/1 -> Compare To Constant2/1
  Constant2/1 -> Switch1/1
  Compare To Constant2/1 -> Switch1/2
  Switch1/1 -> MinMax1/1
  Switch3/1 -> MinMax2/1
  MinMax2/1 -> MinMax Running Resettable1/1
  Constant3/1 -> MinMax Running Resettable/2
  Constant4/1 -> MinMax Running Resettable1/2
  Constant5/1 -> MinMax Running Resettable2/2
  Data Type Conversion/1 -> Disconnection_trigger/1

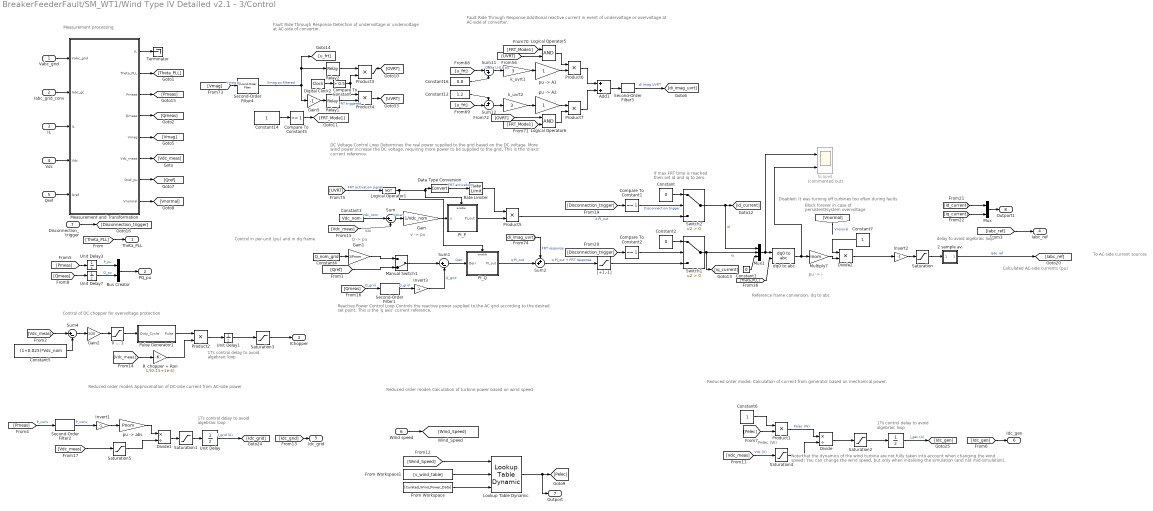
== system BreakerFeederFault/SM_WT1/Wind Type IV Detailed v2.1 - 3/Control ==
  note: Disabled: It was turning off turbines too often during faults
  note: If max FRT time is reached
      | then set id and iq to zero
  note: Measurement processing
  note: Control of DC chopper for overvoltage protection
  note: Fault Ride Through Response
      | Additional reactive current in event of undervoltage or overvoltage at AC-side of converter.
  note: Fault Ride Through Response
      | Detection of undervoltage or undervoltage at AC-side of converter.
  note: Calculated AC-side currents (pu)
  note: pu -> i
  note: Q -> pu
  note: To AC-side current sources
  note: DC Voltage Control Loop
      | Determines the real power supplied to the grid based on the DC voltage. More wind power increase the DC voltage, requiring more power to be supplied to the grid. This is the 'd-axis' current reference.
  note: Reactive Power Control Loop
      | Controls the reactive power supplied to the AC grid according to the desired set point. This is the 'q axis' current reference.
  note: v -> pu
  note: Control in per-unit (pu) and in dq frame
  note: Reference frame conversion: dq to abc
  note: 1Ts control delay to
      | avoid algebraic loop
  note: Reduced order model: Approximation of DC-side current from AC-side power
  note: Reduced order model: Calculation of current from generator based on mechanical power.
  note: delay to avoid
      |  algebraic loop
  note: 1Ts control delay to
      | avoid algebraic loop
  note: Block forever in case of
      | persistent system overvoltage
  note: Reduced order model: Calculation of turbine power based on wind speed
  note: 1Ts control delay to
      | avoid algebraic loop
  note: Note that the dynamics of the wind turbine are not fully taken into account when changing the wind speed! You can change the wind speed, but only when initalising the simulation (and not mid-simulation).
  note: Pelec (W)
  Vabc_grid : Inport
  Iabc_grid_conv : Inport  Port=2
  IL : Inport  Port=3
  Vdc : Inport  Port=4
  Qref : Inport  Port=5
  Wind speed : Inport  Port=6
  Disconnection_trigger : Inport  Port=7
  " " : UnitDelay  SampleTime=-1  HasFrameUpgradeWarning=on
  0 ... 1 : Saturate  UpperLimit=1  LowerLimit=0
  2 sample av. : Subsystem  mask{Init_value=0, Ts=Ts}
      mask prompts: Init_value "Initial value:"; Ts "Sample time (Ts):"
  Add1 : Sum
  Bus Creator : BusCreator  Inputs=2
  Compare To Constant : simulink/Logic and Bit Operations/Compare To Constant  relop=>  const=0.5  OutDataTypeStr=boolean
  Compare To Constant1 : simulink/Logic and Bit Operations/Compare To Constant  relop===  const=1  OutDataTypeStr=boolean
  Compare To Constant2 : simulink/Logic and Bit Operations/Compare To Constant  relop===  const=1  OutDataTypeStr=boolean
  Compare To Constant5 : simulink/Logic and Bit Operations/Compare To Constant  relop===  const=1  OutDataTypeStr=boolean
  Constant : Constant  Value=0
  Constant1 : Constant  Value=0  OutDataTypeStr=Inherit: Inherit via back propagation
  Constant12 : Constant  Value=1.2  SampleTime=Ts
  Constant14 : Constant  SampleTime=Ts
  Constant16 : Constant  Value=0.8  SampleTime=Ts
  Constant2 : Constant  Value=0
  Constant3 : Constant  Value=Vdc_nom
  Constant4 : Constant  Value=Q_nom_grid
  Constant5 : Constant  Value=(1+0.025)*Vdc_nom  SampleTime=Ts
  Constant6 : Constant
  Constant7 : Constant
  Data Type Conversion : DataTypeConversion
  Digital Clock2 : DigitalClock  SampleTime=Ts
  Divide : Product  Inputs=*/
  Divide1 : Product  Inputs=*/
  Divide2 : Product  Inputs=**
  From Workspace : FromWorkspace  VariableName=[Curated_Wind_Power_Data]  SampleTime=0
  From Workspace1 : FromWorkspace  VariableName=[v_wind_table]  SampleTime=0
  Gain : Gain  Gain=1/Vdc_nom
  Gain1 : Gain  Gain=1/Pnom
  Gain2 : Gain  Gain=1/20
  Gain5 : Gain  Gain=-1
  Invert1 : Gain  Gain=-1
  Invert2 : Gain  Gain=-1
  Invert3 : Gain  Gain=-1
  Logical Operator1 : Logic  Operator=NOT  AllPortsSameDT=off  OutDataTypeStr=boolean
  Logical Operator5 : Logic  AllPortsSameDT=off  OutDataTypeStr=boolean
  Logical Operator6 : Logic  AllPortsSameDT=off  OutDataTypeStr=boolean
  Lookup Table Dynamic : simulink/Lookup Tables/Lookup Table Dynamic  LookUpMeth=Interpolation-Use End Values  OutDataType=fixdt('double')  OutScaling=[]  OutputDataTypeScalingMode=Specify via dialog  OutDataTypeStr=double  DoSatur=off
  Manual Switch1 : ManualSwitch  CurrentSetting=0
  Measurement and Transformation : Subsystem
  Multiply7 : Gain  Gain=Inom
  Mux : Mux  Inputs=2
  Mux1 : Mux  Inputs=3
  PI_P : Subsystem
  PI_Q : Subsystem
  Product{1..7} (7 alike) : Product
  Pulse Generator1 : Subsystem  mask{Freq_sawtooth=Freq_sawtooth, Ts=Ts}
      mask prompts: Freq_sawtooth "Frequency of the carrier (sawtooth signal) (Hz):"; Ts "Sample time (Ts) (s):"
  R_chopper + Ron : Gain  Gain=1/(0.15+1e-4)
  Rate Limiter : RateLimiter  RisingSlewLimit=200  FallingSlewLimit=-100  SampleTimeMode=inherited
  Relay1 : Relay  OnSwitchValue=-(0.7)  OffSwitchValue=-(0.8 + 0.05)  OutDataTypeStr=Inherit: Inherit via back propagation
  Relay2 : Relay  OnSwitchValue=1.2 + 0.05  OffSwitchValue=1.2 - 0.05  OutDataTypeStr=Inherit: Inherit via back propagation
  Saturation : Saturate  UpperLimit=1e6  LowerLimit=-1e6
  Saturation1 : Saturate  UpperLimit=1e6  LowerLimit=-1e6
  Saturation2 : Saturate  UpperLimit=1e6  LowerLimit=-1e6
  Saturation3 : Saturate  UpperLimit=10e3  LowerLimit=-10e3
  Saturation4 : Saturate  UpperLimit=1e6  LowerLimit=10
  Saturation5 : Saturate  UpperLimit=1e6  LowerLimit=10
  Scope4 : Scope  Commented=on  NumInputPorts=2
  Second-Order Filter1 : powerlib_meascontrol/Filters/Second-Order Filter  FilterType=Lowpass  Fo=50  Zeta=0.707  Ts=Ts  Initialize=off  Vac_Init="[0,  0,  60]"  Vdc_Init=0  PlotResponse=off  FreqRange=[0, 500, 1]
      settings: SourceProductBaseCode=PS
  Second-Order Filter2 : powerlib_meascontrol/Filters/Second-Order Filter  FilterType=Lowpass  Fo=50  Zeta=0.707  Ts=Ts  Initialize=off  Vac_Init="[0,  0,  60]"  Vdc_Init=0  PlotResponse=off  FreqRange=[0, 500, 1]
      settings: SourceProductBaseCode=PS
  Second-Order Filter3 : powerlib_meascontrol/Filters/Second-Order Filter  FilterType=Lowpass  Fo=1e3  Zeta=0.707  Ts=Ts  Initialize=off  Vac_Init="[0,  0,  60]"  Vdc_Init=0  PlotResponse=off  FreqRange=[0, 500, 1]
      settings: SourceProductBaseCode=PS
  Second-Order Filter4 : powerlib_meascontrol/Filters/Second-Order Filter  FilterType=Lowpass  Fo=100  Zeta=0.707  Ts=Ts  Initialize=off  Vac_Init="[0,  0,  60]"  Vdc_Init=0  PlotResponse=off  FreqRange=[0, 500, 1]
      settings: SourceProductBaseCode=PS
  Sum : Sum  Inputs=|+-
  Sum1 : Sum  Inputs=|+-
  Sum11 : Sum  Inputs=|-+
  Sum12 : Sum  Inputs=+-|
  Sum2 : Sum  Inputs=++|
  Sum4 : Sum  Inputs=|+-
  Switch1 : Switch  Criteria=u2 > Threshold
  Switch2 : Switch  Criteria=u2 > Threshold
  Terminator : Terminator
  Unit Delay : UnitDelay  SampleTime=-1  HasFrameUpgradeWarning=on
  Unit Delay1 : UnitDelay  SampleTime=Ts  HasFrameUpgradeWarning=on
  Unit Delay3 : UnitDelay  SampleTime=Ts  HasFrameUpgradeWarning=on
  Unit Delay7 : UnitDelay  SampleTime=Ts  HasFrameUpgradeWarning=on
  "[+1,-1]" : Saturate  UpperLimit=1  LowerLimit=-1
  dq0 to abc : powerlib_meascontrol/Transformations/dq0 to abc  Alignment=90 degrees behind phase A axis
  k_uvrt1 : Gain  Gain=3
  k_uvrt2 : Gain  Gain=3
  "pu -> A1" : Gain
  "pu -> A2" : Gain
  "pu -> abs" : Gain  Gain=Pnom
  Theta_PLL : Outport  VectorParamsAs1DForOutWhenUnconnected=on
  PQ_pu : Outport  Port=2  VectorParamsAs1DForOutWhenUnconnected=on
  IChopper : Outport  Port=3  VectorParamsAs1DForOutWhenUnconnected=on
  Iabc_ref : Outport  Port=4  VectorParamsAs1DForOutWhenUnconnected=on
  Idc_grid : Outport  Port=5  VectorParamsAs1DForOutWhenUnconnected=on
  Idc_gen : Outport  Port=6  VectorParamsAs1DForOutWhenUnconnected=on
  Outport : Outport  Port=7  VectorParamsAs1DForOutWhenUnconnected=on
  Outport1 : Outport  Port=8  VectorParamsAs1DForOutWhenUnconnected=on
  wires:
  Bus Creator/1 -> PQ_pu/1
  Unit Delay3/1 -> Bus Creator/1  "P_pu"
  Unit Delay7/1 -> Bus Creator/2  "Q_pu"
  [Qmeas] -> Unit Delay7/1
  [Pmeas] -> Unit Delay3/1
  Vdc/1 -> Measurement and Transformation/4(Vdc)
  Measurement and Transformation/1("IL ") -> Terminator/1
  Measurement and Transformation/2(Theta_PLL) -> [Theta_PLL]
  Qref/1 -> Measurement and Transformation/5(Qref)
  IL/1 -> Measurement and Transformation/3(IL)
  Iabc_grid_conv/1 -> Measurement and Transformation/2(Iabc_gc)
  Vabc_grid/1 -> Measurement and Transformation/1(Vabc_grid)
  [Theta_PLL] -> Theta_PLL/1
  Measurement and Transformation/3(Pmeas) -> [Pmeas]
  Measurement and Transformation/4(Qmeas) -> [Qmeas]
  Measurement and Transformation/5(Vmag) -> [Vmag]
  Constant5/1 -> Sum4/2
  [Vdc_meas] -> Sum4/1
  Sum4/1 -> Gain2/1
  Gain2/1 -> 0 ... 1/1
  0 ... 1/1 -> Pulse Generator1/1(Duty_Cycle)
  Measurement and Transformation/6(Vdc_meas) -> [Vdc_meas]
  R_chopper + Ron/1 -> Product2/2
  Product2/1 -> Unit Delay1/1
  [Vdc_meas] -> R_chopper + Ron/1
  Pulse Generator1/1(Pulse) -> Product2/1
  Unit Delay1/1 -> Saturation3/1
  Constant14/1 -> Compare To Constant5/1
  [u_frt] -> Sum11/1
  Compare To Constant5/1 -> [FRT_Mode1]
  Constant12/1 -> Sum12/1
  [u_frt] -> Sum12/2
  [UVRT] -> Logical Operator5/2
  Compare To Constant/1 -> Product4/1, Product3/2
  "pu -> A1"/1 -> Product6/2
  Product7/1 -> Add1/2
  Relay2/1 -> Product3/1
  Product4/1 -> [UVRT]
  Add1/1 -> Second-Order Filter3/1
  Digital Clock2/1 -> Compare To Constant/1
  Product3/1 -> [OVRT]
  Constant16/1 -> Sum11/2
  Second-Order Filter4/1 -> [u_frt], Relay2/1, Gain5/1  "Vmag pu filtered"
  Logical Operator6/1 -> Product7/2
  Sum11/1 -> k_uvrt1/1  "Delta U-0.8 pu"
  Logical Operator5/1 -> Product6/1
  [OVRT] -> Logical Operator6/1
  Gain5/1 -> Relay1/1
  k_uvrt2/1 -> "pu -> A2"/1
  [Vmag] -> Second-Order Filter4/1  "Vmag pu"
  Sum12/1 -> k_uvrt2/1
  [FRT_Mode1] -> Logical Operator6/2
  k_uvrt1/1 -> "pu -> A1"/1
  [FRT_Mode1] -> Logical Operator5/1
  "pu -> A2"/1 -> Product7/1
  Relay1/1 -> Product4/2  "FRT triggered"
  [Qref] -> Manual Switch1/2
  Multiply7/1 -> Divide2/2
  Gain1/1 -> Manual Switch1/1
  Data Type Conversion/1 -> Rate Limiter/1  "FRT activation"
  Constant1/1 -> Mux1/3
  dq0 to abc/1 -> Scope4/2, Multiply7/1
  Manual Switch1/1 -> Sum1/1
  Mux1/1 -> Scope4/1, dq0 to abc/1
  [Vdc_meas] -> Sum/2  "Vdc"
  Invert3/1 -> Sum1/2  "Q_grid"
  Constant3/1 -> Sum/1  "Vdc_nom"
  Sum1/1 -> PI_Q/1(Qerr)  "Qerr"
  [Theta_PLL] -> dq0 to abc/2
  Sum/1 -> Gain/1  "Vdcerr"
  Measurement and Transformation/7(Qref_pu) -> [Qref]
  "pu -> abs"/1 -> Divide1/1
  Invert1/1 -> "pu -> abs"/1
  Divide1/1 -> Saturation1/1
  Unit Delay/1 -> [Idc_grid]  "I_grid (A)"
  Second-Order Filter2/1 -> Invert1/1  "P_conv"
  [Vdc_meas] -> Saturation5/1
  [Idc_grid] -> Idc_grid/1
  Invert2/1 -> Saturation/1
  Saturation3/1 -> IChopper/1
  Second-Order Filter1/1 -> Invert3/1  "Q_grid"
  [Qmeas] -> Second-Order Filter1/1  "Q_grid"
  [Pmeas] -> Second-Order Filter2/1  "P_conv"
  Constant4/1 -> Gain1/1
  Rate Limiter/1 -> Product5/1
  Gain/1 -> PI_P/1(u)
  PI_P/1(PI_out) -> Product5/2
  Saturation/1 -> 2 sample av./1(in)
  Saturation1/1 -> Unit Delay/1
  Saturation5/1 -> Divide1/2
  PI_Q/1(PI_out) -> Sum2/2  "q PI_out"
  Measurement and Transformation/8(Vnormal) -> [Vnormal]
  Divide2/1 -> Invert2/1
  [Vnormal] -> ?  "Vnormal"
  Wind speed/1 -> [Wind_Speed]
  Saturation4/1 -> Divide/2
  Divide/1 -> Saturation2/1
  Saturation2/1 -> " "/1
  [Vdc_meas] -> Saturation4/1  "Vdc (V)"
  Constant6/1 -> Product1/1
  [Idc_gen] -> Idc_gen/1
  [Pelec] -> Product1/2
  Product1/1 -> Divide/1  "Pelec (W)"
  " "/1 -> [Idc_gen]  "I_gen (A)"
  Product6/1 -> Add1/1
  [Iabc_ref] -> Iabc_ref/1
  2 sample av./1(out) -> [Iabc_ref]  "Iabc ref"
  Second-Order Filter3/1 -> [di_imag_uvrt]  "di Imag UVRT"
  Sum2/1 -> "[+1,-1]"/1  "q PI_out + FRT response"
  [di_imag_uvrt] -> Sum2/1  "FRT response"
  [UVRT] -> Logical Operator1/1  "FRT activation signal"
  Logical Operator1/1 -> Data Type Conversion/1, PI_P/Enable, PI_Q/Enable
  Lookup Table Dynamic/1 -> Outport/1, [Pelec]
  [Wind_Speed] -> Lookup Table Dynamic/1
  From Workspace1/1 -> Lookup Table Dynamic/2
  From Workspace/1 -> Lookup Table Dynamic/3
  Switch2/1 -> Mux1/1, [id_current]  "id"
  Switch1/1 -> [iq_current], Mux1/2  "iq"
  Constant/1 -> Switch2/1
  Product5/1 -> Switch2/3  "d PI_out"
  Constant2/1 -> Switch1/1
  "[+1,-1]"/1 -> Switch1/3
  [Disconnection_trigger] -> Compare To Constant1/1
  Compare To Constant1/1 -> Switch2/2  "Disconnection trigger"
  [Disconnection_trigger] -> Compare To Constant2/1
  Compare To Constant2/1 -> Switch1/2
  [id_current] -> Mux/1
  [iq_current] -> Mux/2
  Mux/1 -> Outport1/1
  Disconnection_trigger/1 -> [Disconnection_trigger]
  Constant7/1 -> Divide2/1
